simulink model "problem9"  (R2020a)
settings: Solver=VariableStepAuto  StartTime=0.0  StopTime=10.0  RelTol=1e-3
settings Model: Creator=Jake  LastModifiedBy=Jake

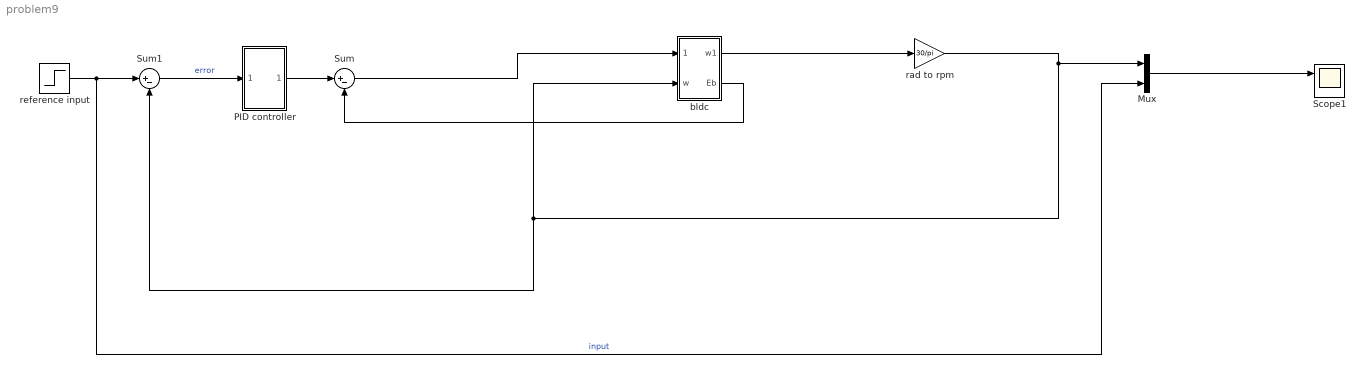
== system problem9 ==
  Mux : Mux  Inputs=2
  PID controller : Subsystem
  Scope1 : Scope  NumInputPorts=2
  Sum : Sum  Inputs=|+-
  Sum1 : Sum  Inputs=|+-
  bldc : Subsystem
  rad to rpm : Gain  Gain=30/pi
  reference input : Step  Time=0  After=1500  SampleTime=0
  wires:
  reference input/1 -> Mux/2, Sum1/1  "input"
  bldc/1(w1) -> rad to rpm/1
  Sum/1 -> bldc/1(In1)
  bldc/2(Eb) -> Sum/2
  Sum1/1 -> PID controller/1(In1)  "error"
  PID controller/1(Out1) -> Sum/1
  rad to rpm/1 -> Mux/1, bldc/2(w), Sum1/2
  Mux/1 -> Scope1/1

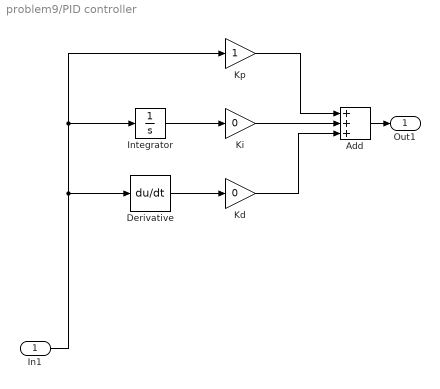
== system problem9/PID controller ==
  In1 : Inport
  Add : Sum  Inputs=+++
  Derivative : Derivative
  Integrator : Integrator
  Kd : Gain  Gain=0
  Ki : Gain  Gain=0
  Kp : Gain
  Out1 : Outport
  wires:
  Kp/1 -> Add/1
  Ki/1 -> Add/2
  Kd/1 -> Add/3
  Derivative/1 -> Kd/1
  Integrator/1 -> Ki/1
  In1/1 -> Derivative/1, Kp/1, Integrator/1
  Add/1 -> Out1/1

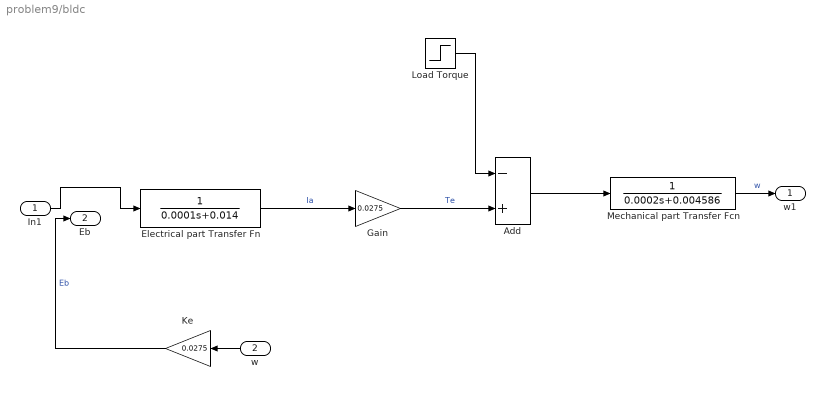
== system problem9/bldc ==
  In1 : Inport
  w : Inport  Port=2
  Add : Sum  Inputs=-+
  Electrical part Transfer Fn : TransferFcn  Denominator=[0.0001 0.014]
  Gain : Gain  Gain=0.0275
  Ke : Gain  Gain=0.0275
  Load Torque : Step  Time=0.1  After=10  SampleTime=0
  Mechanical part Transfer Fcn : TransferFcn  Denominator=[0.0002 0.004586]
  w1 : Outport
  Eb : Outport  Port=2
  wires:
  Gain/1 -> Add/2  "Te"
  w/1 -> Ke/1
  Add/1 -> Mechanical part Transfer Fcn/1
  Load Torque/1 -> Add/1
  In1/1 -> Electrical part Transfer Fn/1
  Ke/1 -> Eb/1  "Eb"
  Electrical part Transfer Fn/1 -> Gain/1  "Ia"
  Mechanical part Transfer Fcn/1 -> w1/1  "w"
